simulink model "Simulation"  (R2022b)
settings: Solver=VariableStepAuto  StartTime=0.0  StopTime=10.0  RelTol=1e-3
PreLoadFcn:
  | InitParams
values from neighbouring files (symbols this model uses):
  CoM = [0, 0, 1.05/2]    [InitParams.m]
  g = [0,0,-9.81]    [InitParams.m]    (also in ParametersFromTVCpaper.m = 9.81)
  massB = 4.2525    [InitParams.m]
  ref_roll = [0,0,1]    [InitParams.m]
  wind = [0,0,2]    [InitParams.m]
libraries: matrix_library x6, aerolibatmos2 x1, sharedtransform x1
settings Model: Creator=nikil  LastModifiedBy=nikil

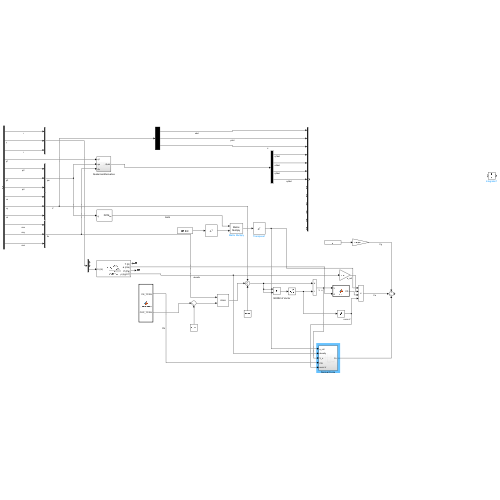
[thumbnail: Simulink's stored preview of the top-level diagram]
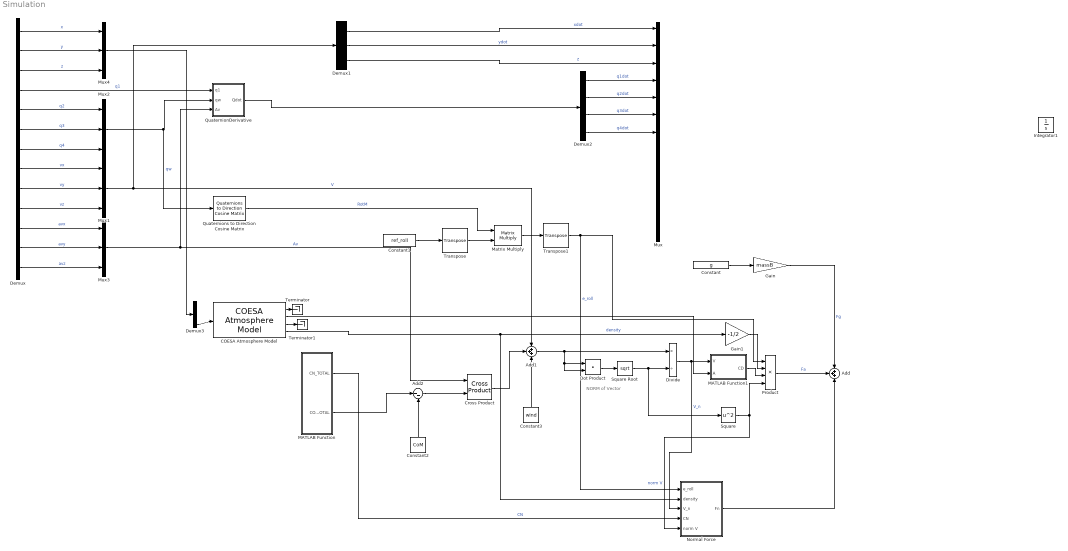
== system Simulation ==
  note: NORM of Vector
  Add : Sum  Inputs=+++
  Add1 : Sum  Inputs=+++
  Add2 : Sum  Inputs=|--
  COESA Atmosphere Model : aerolibatmos2/COESA Atmosphere Model  units=Metric (MKS)  spec=1976 COESA-extended U.S. Standard Atmosphere  model=Profile  profile_var=High temperature  profile_percent=1%  profile_alt=5 km (16404 ft)  envelope_var=High temperature  envelope_percent=1%  action=Warning
  Constant : Constant  Value=g
  Constant1 : Constant  Value=ref_roll
  Constant2 : Constant  Value=CoM
  Constant3 : Constant  Value=wind
  Cross Product : matrix_library/Cross Product
  Demux : Demux  Outputs=13
  Demux1 : Demux  Outputs=3
  Demux2 : Demux
  Demux3 : Demux  Outputs=3
  Divide : Product  Inputs=*/
  Dot Product : DotProduct  OutDataTypeStr=Inherit: Inherit via internal rule
  Gain : Gain  Gain=massB
  Gain1 : Gain  Gain=-1/2
  Integrator1 : Integrator
  MATLAB Function : MATLAB Function  TreatAsAtomicUnit=on
  MATLAB Function1 : MATLAB Function  TreatAsAtomicUnit=on
  Matrix Multiply : Product  Multiplication=Matrix(*)
  Mux : Mux  Inputs=13
  Mux{1..4} (4 alike) : Mux  Inputs=3
  Normal Force : Subsystem
  Product : Product  Inputs=4
  QuaternionDerivative : Subsystem
  Quaternions to Direction Cosine Matrix : sharedtransform/Quaternions to  Direction Cosine Matrix  aMode=aMode
      settings: LibrarySourceBlock=|
      | aerolibtransform2/Quaternions to
      | Direction Cosine Matrix
  Square : Math  Operator=square
  Square Root : Sqrt
  Terminator : Terminator
  Terminator1 : Terminator
  Transpose : matrix_library/Transpose
  Transpose1 : matrix_library/Transpose
  wires:
  Demux/1 -> Mux4/1  "x"
  Demux/3 -> Mux4/3  "z"
  Demux/5 -> Mux2/1  "q2"
  Demux/6 -> Mux2/2  "q3"
  Demux/7 -> Mux2/3  "q4"
  Demux/8 -> Mux1/1  "vx"
  Demux/9 -> Mux1/2  "vy"
  Demux/10 -> Mux1/3  "vz"
  Demux/11 -> Mux3/1  "avx"
  Demux/12 -> Mux3/2  "avy"
  Demux/13 -> Mux3/3  "avz"
  Mux1/1 -> Add1/1, Demux1/1  "V"
  Demux1/1 -> Mux/1  "xdot"
  Demux1/2 -> Mux/2  "ydot"
  Demux1/3 -> Mux/3  "z"
  QuaternionDerivative/1(Qdot) -> Demux2/1
  Demux2/1 -> Mux/4  "q1dot"
  Demux2/2 -> Mux/5  "q2dot"
  Demux2/3 -> Mux/6  "q3dot"
  Demux2/4 -> Mux/7  "q4dot"
  Demux/4 -> QuaternionDerivative/1(q1)  "q1"
  Mux2/1 -> Quaternions to Direction Cosine Matrix/1, QuaternionDerivative/2(qw)  "qw"
  Mux3/1 -> Cross Product/1, QuaternionDerivative/3(Av)  "Av"
  Demux/2 -> Mux4/2  "y"
  Constant/1 -> Gain/1
  Gain/1 -> Add/1  "Fg"
  Quaternions to Direction Cosine Matrix/1 -> Matrix Multiply/1  "RotM"
  Constant1/1 -> Transpose/1
  Transpose/1 -> Matrix Multiply/2
  Matrix Multiply/1 -> Transpose1/1
  Mux4/1 -> Demux3/1
  Demux3/3 -> COESA Atmosphere Model/1
  COESA Atmosphere Model/1 -> Terminator/1
  COESA Atmosphere Model/3 -> Terminator1/1
  Constant2/1 -> Add2/2
  MATLAB Function/2(COP_TOTAL) -> Add2/1
  Add2/1 -> Cross Product/2
  Cross Product/1 -> Add1/2
  Constant3/1 -> Add1/3
  Add1/1 -> Dot Product/2, Dot Product/1, Divide/1
  Dot Product/1 -> Square Root/1
  Square Root/1 -> Square/1, Divide/2
  Divide/1 -> Normal Force/3(V_n), MATLAB Function1/1(V)  "V_n"
  COESA Atmosphere Model/2 -> MATLAB Function1/2(A)
  Gain1/1 -> Product/2
  COESA Atmosphere Model/4 -> Normal Force/2(density), Gain1/1  "density"
  MATLAB Function1/1(CD) -> Product/3
  Square/1 -> Normal Force/5(norm V), Product/4  "norm V"
  Transpose1/1 -> Normal Force/1(e_roll), Product/1  "e_roll"
  Product/1 -> Add/2  "Fa"
  MATLAB Function/1(CN_TOTAL) -> Normal Force/4(CN)  "CN"
  Normal Force/1(Fn) -> Add/3

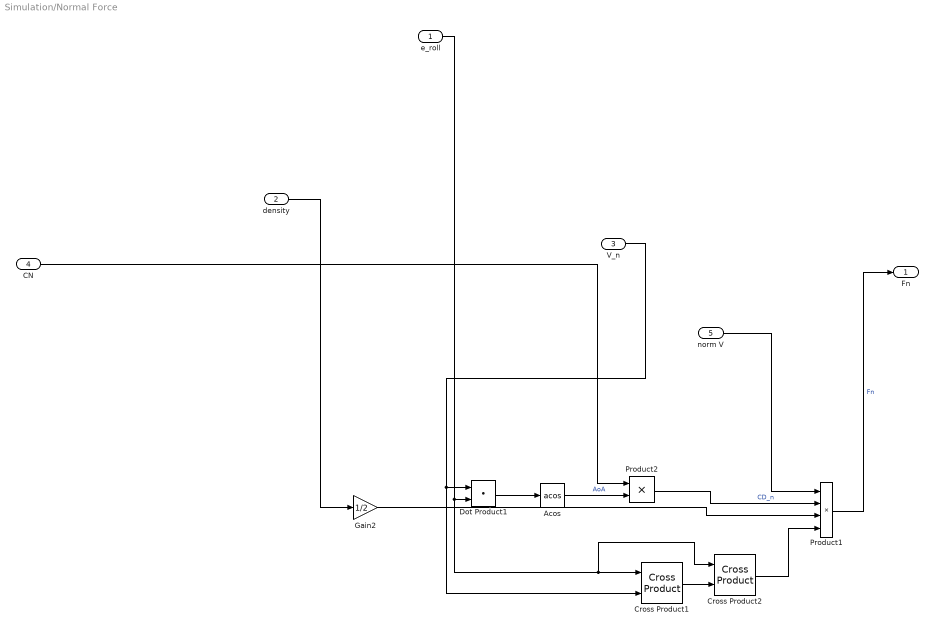
== system Simulation/Normal Force ==
  e_roll : Inport
  density : Inport  Port=2
  V_n : Inport  Port=3
  CN : Inport  Port=4
  norm V : Inport  Port=5
  Acos : Trigonometry  Operator=acos
  Cross Product1 : matrix_library/Cross Product
  Cross Product2 : matrix_library/Cross Product
  Dot Product1 : DotProduct  OutDataTypeStr=Inherit: Inherit via internal rule
  Gain2 : Gain  Gain=1/2
  Product1 : Product  Inputs=4
  Product2 : Product
  Fn : Outport
  wires:
  norm V/1 -> Product1/1
  e_roll/1 -> Cross Product2/1, Cross Product1/1, Dot Product1/2
  Product2/1 -> Product1/2  "CD_n"
  Cross Product2/1 -> Product1/4
  Acos/1 -> Product2/2  "AoA"
  Cross Product1/1 -> Cross Product2/2
  V_n/1 -> Cross Product1/2, Dot Product1/1
  Gain2/1 -> Product1/3
  Dot Product1/1 -> Acos/1
  density/1 -> Gain2/1
  CN/1 -> Product2/1
  Product1/1 -> Fn/1  "Fn"

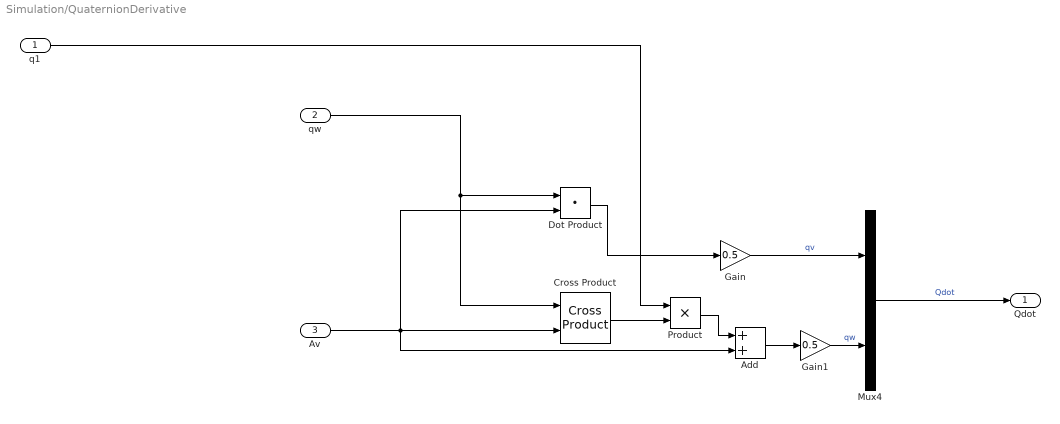
== system Simulation/QuaternionDerivative ==
  q1 : Inport
  qw : Inport  Port=2
  Av : Inport  Port=3
  Add : Sum
  Cross Product : matrix_library/Cross Product
  Dot Product : DotProduct  OutDataTypeStr=Inherit: Inherit via internal rule
  Gain : Gain  Gain=0.5
  Gain1 : Gain  Gain=0.5
  Mux4 : Mux  Inputs=2
  Product : Product
  Qdot : Outport
  wires:
  qw/1 -> Cross Product/1, Dot Product/1
  Av/1 -> Add/2, Dot Product/2, Cross Product/2
  Dot Product/1 -> Gain/1
  Gain/1 -> Mux4/1  "qv"
  q1/1 -> Product/1
  Gain1/1 -> Mux4/2  "qw"
  Product/1 -> Add/1
  Mux4/1 -> Qdot/1  "Qdot"
  Cross Product/1 -> Product/2
  Add/1 -> Gain1/1

== matlab function Simulation/MATLAB Function ==
  data: CN_TOTAL output; COP_TOTAL output
function [CN_TOTAL, COP_TOTAL] = coefficients()
% Normal force coeff for body, fins, nosecone (per radian)
CN_NOSE = 2;
CN_BODY = 0;
CN_FINS = 16*(HEIGHT_FIN/DIAMETER_BODY)^2 / (1 + sqrt(1 + (2*MIDCHORD_FIN / (ROOTCHORD_FIN + TIPCHORD_FIN))^2));
%correction 
K = 1  +TIPCHORD_FIN/(HEIGHT_FIN + TIPCHORD_FIN);
CN_INTERFERENCE = K*CN_FINS;
CN_TOTAL = CN_INTERFERENCE + CN_BODY + CN_NOSE + CN_FINS;



% COP calculation
COP_NOSE = 0.466.*[0, 0, LEN_NOSECONE]; %Vertical vec for now 
%relative to tip CHORD
COP_FINS_TIP = (SWEEPLENGTH_FIN/3) * ((ROOTCHORD_FIN + 2*TIPCHORD_FIN) / (ROOTCHORD_FIN + TIPCHORD_FIN)) + ...
                (1/6)*(ROOTCHORD_FIN + TIPCHORD_FIN - (ROOTCHORD_FIN*TIPCHORD_FIN)/(ROOTCHORD_FIN + TIPCHORD_FIN));

COP_FINS = [0,0,COP_FINS_TIP+(LEN_ROCKET-ROOTCHORD_FIN)]; %from nose cone
COP_INTERFERENCE = [0,0,LEN_ROCKET-ROOTCHORD_FIN]; %from nose cone

COP_TOTAL = (COP_INTERFERENCE.*CN_INTERFERENCE + COP_FINS.*CN_FINS + COP_NOSE.*CN_NOSE)/CN_TOTAL; %FROM NOSE TIP

== matlab function Simulation/MATLAB Function1 ==
  data: V input; CD output; A input
function CD  = fcn(V,A)
% drag force coeff for body, fins, nosecone 
% FROM MANDEL'S TOPICS IN ADVANCED ROCKETRY (PG 447)
Re_B = V .* LEN_ROCKET./KINEMATIC_VISC;
%B = 5*10^5*(0.73/Re_B^(1/5) - 1.328/sqrt(Re_B));
% if Re_B > 5*10^5
%     SKINFRICTION_BODY = 0.073/Re_B^(1/5) - B/Re_B;
% else
    SKINFRICTION_BODY = 0.073./Re_B.^(1/5);
% end 
AREA_RATIO = 4*(LEN_ROCKET-LEN_NOSECONE)/DIAMETER_BODY + 2.7*LEN_NOSECONE/DIAMETER_BODY;
F = 1 + 60/(LEN_ROCKET/DIAMETER_BODY)^3 + 0.0025*LEN_ROCKET/DIAMETER_BODY;
CD_FB = SKINFRICTION_BODY.*F.*AREA_RATIO; %forbody body drag
CD_DB = 0.029*(1/1)^3./sqrt(CD_FB); %forbody base drag
Re_F = V .* AVERAGECHORD_FIN ./ KINEMATIC_VISC;
SKINFRICTION_FIN = 1.328./sqrt(Re_F);
TC_RATIO = THICKNESS_FIN / AVERAGECHORD_FIN;
CD_F = 2.*SKINFRICTION_FIN.*(1+2*TC_RATIO).*AREA_FIN./AREA_FRONTBODY;
Ma = V./A;

if(Ma<1)
    CD = (CD_F + CD_DB + CD_FB).*(1./sqrt(1 - Ma.^2));
else
    CD = (CD_F + CD_DB + CD_FB).*(1./sqrt(Ma.^2 - 1));
end
